simulink model "exp2_p2"  (R2018a)
settings: Solver=VariableStepAuto  StartTime=0.0  StopTime=10.0  RelTol=1e-3
libraries: powerlib x10, powerlib_meascontrol x3
settings Model: Creator=Administrator  LastModifiedBy=Administrator

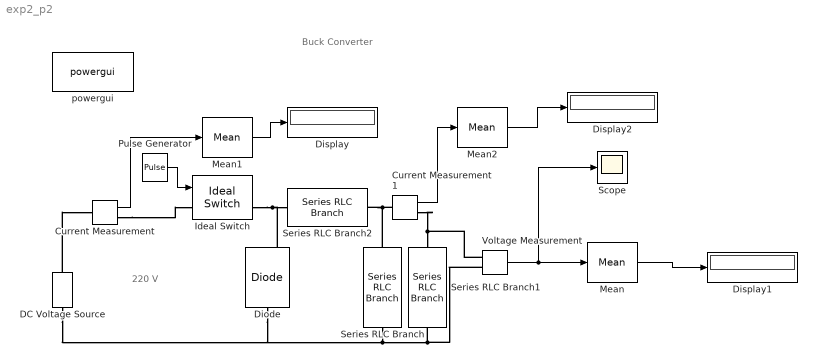
== system exp2_p2 ==
  note: 220 V
  note: Buck Converter
  Current Measurement : powerlib/Measurements/Current Measurement  PhasorSimulation=off  OutputType=Complex  PSBequivalent=0
  Current Measurement1 : powerlib/Measurements/Current Measurement  PhasorSimulation=off  OutputType=Complex  PSBequivalent=0
  DC Voltage Source : powerlib/Electrical Sources/DC Voltage Source  Amplitude=220  Measurements=None
  Diode : powerlib/Power Electronics/Diode  Ron=0.001  Lon=0  Vf=0.8  IC=0  UseSnubber=0  Rs=500  Cs=250e-9  Measurements=on
  Display : Display
  Display1 : Display
  Display2 : Display
  Ideal Switch : powerlib/Power Electronics/Ideal Switch  Ron=0.001  Lon=0  IC=0  Rs=1e5  Cs=inf  Measurements=on
  Mean : powerlib_meascontrol/Measurements/Mean  Freq=10000  Vinit=0  Ts=0
  Mean1 : powerlib_meascontrol/Measurements/Mean  Freq=10000  Vinit=0  Ts=0
  Mean2 : powerlib_meascontrol/Measurements/Mean  Freq=10000  Vinit=0  Ts=0
  Pulse Generator : DiscretePulseGenerator  PulseType=Time based  Period=1/10000  PulseWidth=50
  Scope : Scope
  Series RLC Branch : powerlib/Elements/Series RLC Branch  LConnTagsString=__new0  RConnTagsString=__new0  BranchType=C  Resistance=1  Inductance=1e-3  SetiL0=off  InitialCurrent=0  Capacitance=100*1e-6  Setx0=off  InitialVoltage=0  Measurements=None
  Series RLC Branch1 : powerlib/Elements/Series RLC Branch  LConnTagsString=__new0  RConnTagsString=__new0  BranchType=R  Resistance=22  Inductance=1e-3  SetiL0=off  InitialCurrent=0  Capacitance=1e-6  Setx0=off  InitialVoltage=0  Measurements=None
  Series RLC Branch2 : powerlib/Elements/Series RLC Branch  LConnTagsString=__new0  RConnTagsString=__new0  BranchType=L  Resistance=1  Inductance=100*1e-3  SetiL0=off  InitialCurrent=0  Capacitance=1e-6  Setx0=off  InitialVoltage=0  Measurements=None
  Voltage Measurement : powerlib/Measurements/Voltage Measurement  PhasorSimulation=off  OutputType=Complex  PSBequivalent=0
  powergui : powerlib/powergui  Priority=1  SimulationMode=Continuous  SampleTime=50e-6  frequency=60  Iterations=50  frequencyindice=0  Pbase=100e6  ErrMax=1e-4  UnitsV=kV  UnitsW=MW  buscounter=0  FunctionMessages=off  echomessages=off  EnableUseOfTLC=off  CurrentSourceSwitches=off  DisableSnubberDevices=off  DisableRonSwitches=off  DisableVfSwitches=off  DisplayEquations=off  SolverType=Tustin/Backward Euler (TBE)  Interpol=off  ExternalGateDelay=off  methode=off  Ts=100  x0status=zero  SPID=on  SwTol=0  HookPort=off  RestoreLinks=warning  ResistiveCurrentMeasurement=off  Frange=[0:2:500]  Ylog=off  Xlog=on  ShowGrid=off  save=off  variable=ZData  structure=0  ZoomFFT=off  StartTime=0.0  cycles=1  DisplayStyle=1  fundamental=60  FreqAxis=off  MaxFrequency=1000  frequencyindicesteady=1  RmsSteady=1  display=off
  wires:
  Mean/1 -> Display1/1
  Voltage Measurement/1 -> Scope/1, Mean/1
  Pulse Generator/1 -> Ideal Switch/1
  Mean1/1 -> Display/1
  Current Measurement1/1 -> Mean2/1
  Mean2/1 -> Display2/1
  Current Measurement/1 -> Mean1/1
  connections:
  Current Measurement1/RConn1 -- Voltage Measurement/LConn1 -- Series RLC Branch1/LConn1
  Voltage Measurement/LConn2 -- Diode/LConn1 -- DC Voltage Source/LConn1 -- Series RLC Branch/RConn1 -- Series RLC Branch1/RConn1
  DC Voltage Source/RConn1 -- Current Measurement/LConn1
  Ideal Switch/RConn1 -- Diode/RConn1 -- Series RLC Branch2/LConn1
  Current Measurement/RConn1 -- Ideal Switch/LConn1
  Series RLC Branch/LConn1 -- Current Measurement1/LConn1 -- Series RLC Branch2/RConn1
